simulink model "IKTrajectoryControlExample"  (R2020a)
settings: Solver=FixedStepAuto  StartTime=0.0  StopTime=40  FixedStep=Ts  RelTol=1e-3
PostLoadFcn:
  | sawyer = importrobot('sawyer.urdf');
  | sawyer.DataFormat = 'column';
  | 
  | I = imread('coins.png');
  | imageOrigin = [0.4,0.2,0.08];
  | scale = .0015;
model workspace (MAT data in the model file):
  filterConst = 0.08
values from neighbouring files (symbols this model uses):
  q0 = [0.422405030328 0 -1.22880122279 -0.410622116121 2.12106389544 0.20550569385 0.715545052926 1.62245604003]    [defaultTrajControlSLXParams.mat]
  wayPoints = [0.4 0.4 0.4 0.4 0.4 0.4 0.4 0.4 0.4 0.4 0.4 0.4 ... (3426 elements, 571x6)]    [defaultTrajControlSLXParams.mat]
  weights = [1 1 1 1 1 1]    [defaultTrajControlSLXParams.mat]
undefined symbols (not defined in the file or in its folder): Levenberg, Marquardt
libraries: robotmaniplib x6, simulink x3
settings Model: OrderedModelArguments=off  Creator=The MathWorks, Inc.  LastModifiedBy=The MathWorks, Inc.
settings DataIOCC: SaveFormat=Array  ReturnWorkspaceOutputs=off
settings DebuggingCC: PregeneratedLibrarySubsystemCodeDiagnostic=none  ArithmeticOperatorsInVariantConditions=warning
settings SFSimCC: SimUseLocalCustomCode=off  CustomCodeUndefinedFunction=UseInterfaceOnly
settings RTWCC: RTWUseLocalCustomCode=off

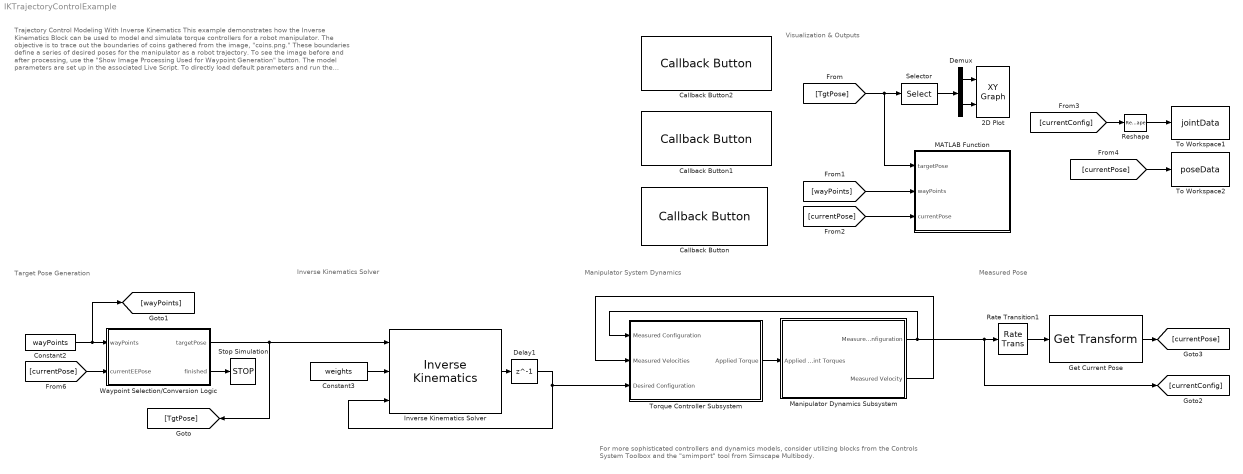
== system IKTrajectoryControlExample ==
  note: Visualization & Outputs
  note: Trajectory Control Modeling With Inverse Kinematics
      | This example demonstrates how the Inverse Kinematics Block can be used to model and simulate torque controllers for a robot manipulator.
      |
      | The objective is to trace out the boundaries of coins gathered from the image, "coins.png." These boundaries define a series of desired poses for the manipulator as a robot trajectory. To see the image before and after processing, use the "Show Image Processing Used for Waypoint Generation" button.
      |
      | The model parameters are set up in the associated Live Script. To directly load default parameters and run the model, click the "Load Default Parameters" button and simulate. Please be aware that this will overwrite any existing variables in the MATLAB workspace.
      |
      | The trajectory is specified in the wayPoints matrix, where each waypoint is a six-element vector specifing [X Y Z] coordinates and [Z Y X] euler angles for the end effector of the manipulator. These waypoints are converted into a vector of desired joint configurations using inverse kinematics. The desired joint configurations are fed to a controller that generates the torques necessary to drive the arm along the trajectory.
      |
      | To visualize the motion of the entire manipulator, use the "Visualize Model Output with Manipulator Mesh" button after simulation.
      |
      | © Copyright 2018-2019 The MathWorks, Inc.
  note: Measured Pose
  note: Inverse Kinematics Solver
  note: Manipulator System Dynamics
  note: Target Pose Generation
  note: For more sophisticated controllers and dynamics models, consider utilizing blocks from the Controls System Toolbox and the "smimport" tool from Simscape Multibody.
  2D Plot : simulink/Sinks/XY Graph  xmin=.2  xmax=.9  ymin=0  ymax=.7  st=-1
  Callback Button : CallbackButton  ButtonText=Show Image Processing Used for Waypoint Generation
      settings: ClickFcn=|
      | f1 = figure(1);
      | f1.Position = [158 253 953 335];
      | I1 = imread('coins.png');
      | I2 = imread('coinBoundaries.png');
      | 
      | subplot(1,2,1)
      | imshow(I1, 'Border', 'tight')
      | title('Original Image')
      | 
      | subplot(1,2,2)
      | imshow(I2, 'Border', 'tight')
      | title('Processed Image with Boundary Detection')
  Callback Button1 : CallbackButton  ButtonText=Visualize Model Output with Manipulator Mesh
      settings: ClickFcn=|
      | if exist('jointData', 'var')
      |     exampleHelperVisualizeIK(I, jointData, poseData, sawyer, imageOrigin, scale);
      | else
      |     sim(gcs)
      |     exampleHelperVisualizeIK(I, jointData, poseData, sawyer, imageOrigin, scale);
      | end
  Callback Button2 : CallbackButton  ButtonText=Load Default Parameters (will overwrite workspace)
      settings: ClickFcn=load defaultTrajControlSLXParams.mat
  Constant2 : Constant  Value=wayPoints
  Constant3 : Constant  Value=weights
  Delay1 : Delay  DelayLength=1  InitialCondition=q0
  Demux : Demux  Outputs=2
  Get Current Pose : robotmaniplib/Get Transform  RigidBodyTree=sawyer  SourceBody=right_hand  TargetBody=base  SimulateUsing=Interpreted execution
  Inverse Kinematics Solver : robotmaniplib/Inverse Kinematics  RigidBodyTree=sawyer  EndEffector=right_hand  ShowInfo=off  SolverName=Levenberg-Marquardt  EnforceJointLimits=on  MaxIterations=1500  MaxTime=10  GradientTolerance=1e-7  SolutionTolerance=1e-5  StepTolerance=1e-14  ErrorChangeTolerance=1e-8  UseErrorDamping=on  DampingBias=0.0025  SimulateUsing=Interpreted execution
  MATLAB Function : MATLAB Function  TreatAsAtomicUnit=on  SystemSampleTime=.1
  Manipulator Dynamics Subsystem : Subsystem
  Rate Transition1 : RateTransition
  Reshape : Reshape
  Selector : Selector  NumberOfDimensions=2  IndexOptions=Index vector (dialog),Index vector (dialog)  Indices=[1 2],4  OutputSizes=1,1
  Stop Simulation : Stop
  To Workspace1 : ToWorkspace  VariableName=jointData  SampleTime=-1
      settings: Save2DSignal=2-D array (concatenate along first dimension)
  To Workspace2 : ToWorkspace  VariableName=poseData  SampleTime=-1
  Torque Controller Subsystem : Subsystem
  Waypoint Selection/Conversion Logic : Stateflow chart  TreatAsAtomicUnit=on
  wires:
  Constant2/1 -> [wayPoints], Waypoint Selection/Conversion Logic/1(wayPoints)
  Rate Transition1/1 -> Get Current Pose/1
  Get Current Pose/1 -> [currentPose]
  Torque Controller Subsystem/1(Applied Torque) -> Manipulator Dynamics Subsystem/1(Applied Joint Torques)
  Manipulator Dynamics Subsystem/1(Measured Configuration) -> Torque Controller Subsystem/1(Measured Configuration), [currentConfig], Rate Transition1/1
  Manipulator Dynamics Subsystem/2(Measured Velocity) -> Torque Controller Subsystem/2(Measured Velocities)
  Delay1/1 -> Inverse Kinematics Solver/3, Torque Controller Subsystem/3(Desired Configuration)
  Waypoint Selection/Conversion Logic/2(finished) -> Stop Simulation/1
  Constant3/1 -> Inverse Kinematics Solver/2
  Waypoint Selection/Conversion Logic/1(targetPose) -> [TgtPose], Inverse Kinematics Solver/1
  Inverse Kinematics Solver/1 -> Delay1/1
  Selector/1 -> Demux/1
  Demux/1 -> 2D Plot/1
  Demux/2 -> 2D Plot/2
  [TgtPose] -> Selector/1, MATLAB Function/1(targetPose)
  [wayPoints] -> MATLAB Function/2(wayPoints)
  [currentPose] -> MATLAB Function/3(currentPose)
  [currentPose] -> Waypoint Selection/Conversion Logic/2(currentEEPose)
  [currentConfig] -> Reshape/1
  [currentPose] -> To Workspace2/1
  Reshape/1 -> To Workspace1/1

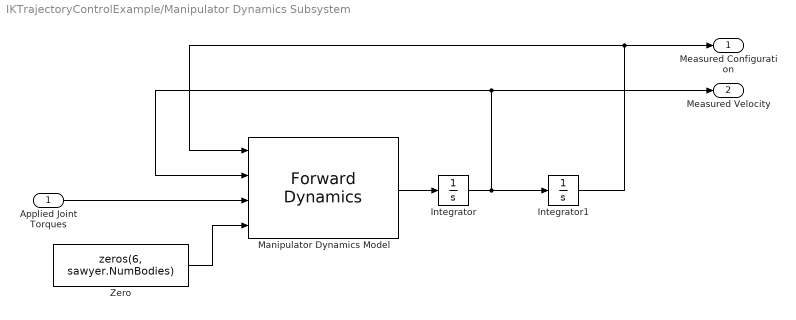
== system IKTrajectoryControlExample/Manipulator Dynamics Subsystem ==
  Applied Joint Torques : Inport
  Integrator : Integrator
  Integrator1 : Integrator  InitialCondition=q0
  Manipulator Dynamics Model : robotmaniplib/Forward Dynamics  RigidBodyTree=sawyer  SimulateUsing=Interpreted execution
  Zero : Constant  Value=zeros(6, sawyer.NumBodies)  OutDataTypeStr=Inherit: Inherit via back propagation
  Measured Configuration : Outport  VectorParamsAs1DForOutWhenUnconnected=off
  Measured Velocity : Outport  Port=2  VectorParamsAs1DForOutWhenUnconnected=off
  wires:
  Integrator1/1 -> Manipulator Dynamics Model/1, Measured Configuration/1
  Manipulator Dynamics Model/1 -> Integrator/1
  Integrator/1 -> Integrator1/1, Manipulator Dynamics Model/2, Measured Velocity/1
  Applied Joint Torques/1 -> Manipulator Dynamics Model/3
  Zero/1 -> Manipulator Dynamics Model/4

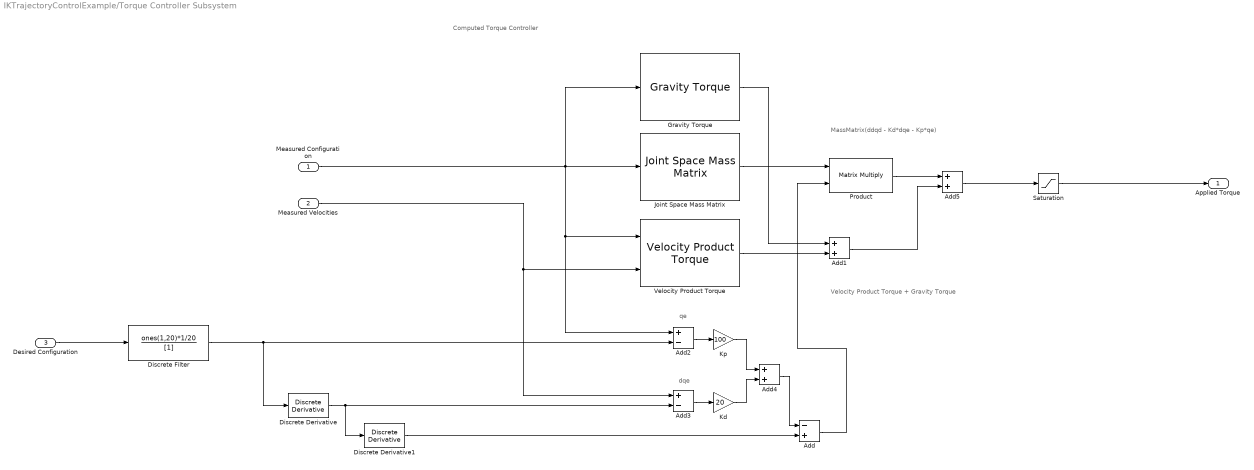
== system IKTrajectoryControlExample/Torque Controller Subsystem ==
  note: Computed Torque Controller
  note: MassMatrix(ddqd - Kd*dqe - Kp*qe)
  note: Velocity Product Torque + Gravity Torque
  note: dqe
  note: qe
  Measured Configuration : Inport
  Measured Velocities : Inport  Port=2
  Desired Configuration : Inport  Port=3
  Add : Sum  Inputs=-+
  Add1 : Sum
  Add2 : Sum  Inputs=+-
  Add3 : Sum  Inputs=+-
  Add4 : Sum
  Add5 : Sum
  Discrete Derivative : simulink/Discrete/Discrete Derivative  gainval=1.0  ICPrevScaledInput=0.0  OutMin=[]  OutMax=[]  OutDataType=fixdt(1, 16)  OutScaling=2^-10  DoSatur=off
  Discrete Derivative1 : simulink/Discrete/Discrete Derivative  gainval=1.0  ICPrevScaledInput=0.0  OutMin=[]  OutMax=[]  OutDataType=fixdt(1, 16)  OutScaling=2^-10  DoSatur=off
  Discrete Filter : DiscreteFilter  Numerator=ones(1,20)*1/20  Denominator=[1]  InitialStates=repmat(q0',19,1)
  Gravity Torque : robotmaniplib/Gravity Torque  RigidBodyTree=sawyer  SimulateUsing=Interpreted execution
  Joint Space Mass Matrix : robotmaniplib/Joint Space Mass Matrix  RigidBodyTree=sawyer  SimulateUsing=Interpreted execution
  Kd : Gain  Gain=20
  Kp : Gain  Gain=100
  Product : Product  Multiplication=Matrix(*)
  Saturation : Saturate  UpperLimit=100  LowerLimit=-100
  Velocity Product Torque : robotmaniplib/Velocity Product Torque  RigidBodyTree=sawyer  SimulateUsing=Interpreted execution
      settings: SourceProductBaseCode=RO
  Applied Torque : Outport  VectorParamsAs1DForOutWhenUnconnected=off
  wires:
  Saturation/1 -> Applied Torque/1
  Velocity Product Torque/1 -> Add1/2
  Gravity Torque/1 -> Add1/1
  Add1/1 -> Add5/2
  Product/1 -> Add5/1
  Add5/1 -> Saturation/1
  Kd/1 -> Add4/2
  Kp/1 -> Add4/1
  Add3/1 -> Kd/1
  Add2/1 -> Kp/1
  Discrete Derivative/1 -> Add3/2, Discrete Derivative1/1
  Desired Configuration/1 -> Discrete Filter/1
  Add/1 -> Product/2
  Discrete Derivative1/1 -> Add/2
  Add4/1 -> Add/1
  Measured Velocities/1 -> Velocity Product Torque/2, Add3/1
  Measured Configuration/1 -> Add2/1, Velocity Product Torque/1, Gravity Torque/1, Joint Space Mass Matrix/1
  Joint Space Mass Matrix/1 -> Product/1
  Discrete Filter/1 -> Discrete Derivative/1, Add2/2

== matlab function IKTrajectoryControlExample/MATLAB Function ==
  data: targetPose input; wayPoints input; currentPose input
function waypointTracking(targetPose, wayPoints, currentPose)
%#codegen

persistent f a

if isempty(f)
    f = figure;
    title('Waypoint Tracking');
    a = axes;
    axis(a, [	0.4,0.8, 0.2,0.635, 0.05,0.3]);
    set(f, 'Visible', 'on');
end

targetPoint = targetPose(1:3,end);
currentPoint = currentPose(1:3,end);

plot3(a,wayPoints(:,1), wayPoints(:,2), wayPoints(:,3), 'b.', 'MarkerSize', 1);
hold on
plot3(a,targetPoint(1), targetPoint(2), targetPoint(3), 'go', 'MarkerSize', 5);
plot3(a,currentPoint(1), currentPoint(2), currentPoint(3), 'ro', 'MarkerSize', 5);

hold off

== stateflow chart IKTrajectoryControlExample/Waypoint Selection//Conversion Logic ==
  (default) -> (junction 1) : %Check EE deviation from Target Pose
      | {error = vecnorm(targetPose(1:3, :) - currentEEPose(1:3, :), 2, 1); }
  (junction 1) -> (junction 3) [order 1] : [all(error < tol )]
  (junction 3) -> (junction 19) [order 1] : [index == length(wayPoints)]
  (junction 1) -> (junction 5) [order 2]
  (junction 3) -> (junction 7) [order 2] : %Select next Waypoint
      | {index = index + 1;}
  (junction 19) -> (junction 22) : %Stop Simulation
      | {finished = true;}
  (junction 7) -> (junction 5)
  (junction 22) -> (junction 7)
  (junction 5) -> (junction 10) : %Update Target and Convert to Homogenous Transform
      | { targetPose = eul2tform(wayPoints(index,4:6));
      | targetPose(1:3,end) = wayPoints(index,1:3)'; }
  data: targetPose output =initTargetPose; wayPoints input; currentEEPose input; finished output =false; index local [..length(wayPoints)] =1; tol local =.01; error local
